simulink model "CA_2"  (Simulink 6.6)
settings: Solver=ode45  StartTime=0.0  StopTime=18e-6  RelTol=1e-3
libraries: commseqgen2 x1, commutil2 x1
settings Model: Creator=Мама Люда  LastModifiedBy=Мама Люда

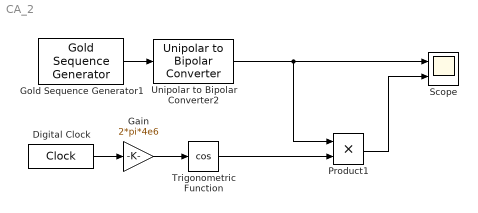
== system CA_2 ==
  Digital Clock : DigitalClock  SampleTime=1e-8
  Gain : Gain  Gain=2*pi*4e6
  Gold Sequence Generator1 : commseqgen2/Gold Sequence Generator  SystemSampleTime=-1  genPoly1=[1 0 0 1 0 0 0 0 0 0 1]  iniState1=[1 1 1 1 1 1 1 1 1 1]  genPoly2="[1 0 1 1 0  0 1 0 1 1 1]"  iniState2=[1 1 1 1 1 1 1 1 1 1]  index=0  shift=0  ts=0.9775e-6  frameBased=off  sampPerFrame=1  reset=off  outDataType=double
  Product1 : Product  RndMeth=Zero
  Scope : Scope  NumInputPorts=2
      settings: TimeRange=4e-005  YMin=-2~-2  YMax=2~2  SampleInput=on  SampleTime=1e-8
  Trigonometric Function : Trigonometry  Operator=cos
  Unipolar to Bipolar Converter2 : commutil2/Unipolar to Bipolar Converter  SystemSampleTime=-1  M=2  polarity=Positive  dataType=double
  wires:
  Gold Sequence Generator1/1 -> Unipolar to Bipolar Converter2/1
  Unipolar to Bipolar Converter2/1 -> Scope/1, Product1/1
  Digital Clock/1 -> Gain/1
  Gain/1 -> Trigonometric Function/1
  Trigonometric Function/1 -> Product1/2
  Product1/1 -> Scope/2
